simulink library "casper_library_scopes"  (Simulink 7.4)
settings: Solver=ode45  SolverMode=SingleTasking  StartTime=0.0  StopTime=10.0  RelTol=1e-3
libraries: xbsIndex_r4 x369, xps_library x28, casper_library_misc x12, casper_library_scopes x4, simulink x1
(part 2 of 4)

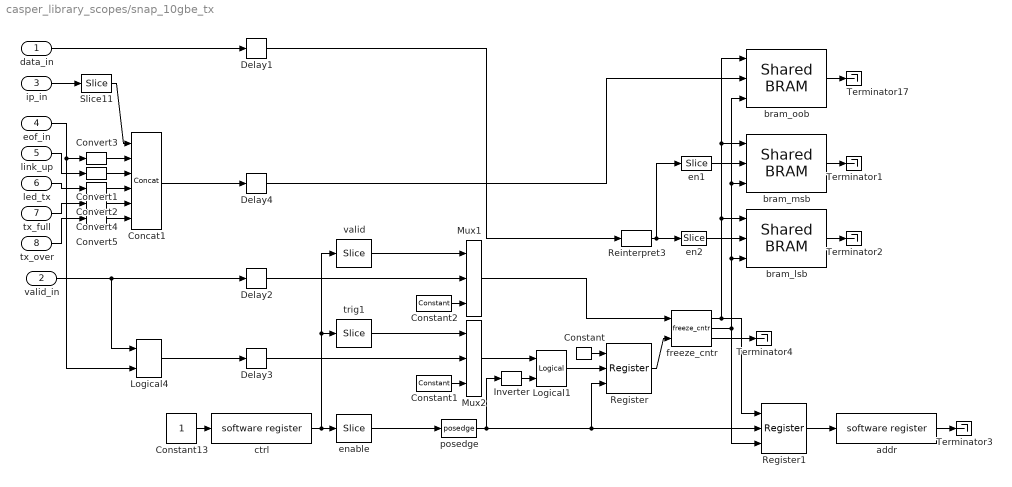
== system casper_library_scopes/snap_10gbe_tx ==
  data_in : Inport  OutDataType=sfix(16)  OutScaling=2^0
  valid_in : Inport  Port=2  OutDataType=sfix(16)  OutScaling=2^0
  ip_in : Inport  Port=3  OutDataType=sfix(16)  OutScaling=2^0
  eof_in : Inport  Port=4  OutDataType=sfix(16)  OutScaling=2^0
  link_up : Inport  Port=5  OutDataType=sfix(16)  OutScaling=2^0
  led_tx : Inport  Port=6  OutDataType=sfix(16)  OutScaling=2^0
  tx_full : Inport  Port=7  OutDataType=sfix(16)  OutScaling=2^0
  tx_over : Inport  Port=8  OutDataType=sfix(16)  OutScaling=2^0
  Concat1 : xbsIndex_r4/Concat  num_inputs=6  dbl_ovrd=off  block_type=concat
      settings: block_version=10.1.3
  Constant : xbsIndex_r4/Constant  arith_type=Boolean  const=1  n_bits=1  bin_pt=0  explicit_period=on  period=1  equ=P=C  opselect=C  inp2=PCIN>>17  opr=+  inp1=P  carry=CIN  dbl_ovrd=off  block_type=constant
  Constant1 : xbsIndex_r4/Constant  arith_type=Boolean  const=1  n_bits=1  bin_pt=0  explicit_period=on  period=1  equ=P=C  opselect=C  inp2=PCIN>>17  opr=+  inp1=P  carry=CIN  dbl_ovrd=off  block_type=constant
  Constant13 : Constant  OutDataType=sfix(16)  OutScaling=2^0
  Constant2 : xbsIndex_r4/Constant  arith_type=Boolean  const=1  n_bits=1  bin_pt=0  explicit_period=on  period=1  equ=P=C  opselect=C  inp2=PCIN>>17  opr=+  inp1=P  carry=CIN  dbl_ovrd=off  block_type=constant
  Convert{1..5} (5 alike) : xbsIndex_r4/Convert  arith_type=Unsigned  n_bits=1  bin_pt=0  quantization=Truncate  overflow=Wrap  latency=0  dbl_ovrd=off  pipeline=off  block_type=convert
      settings: xl_area=[0, 0, 0, 0, 0, 0, 0]  block_version=10.1.3
  Delay{1..4} (4 alike) : xbsIndex_r4/Delay  en=off  latency=2  dbl_ovrd=off  reg_retiming=on  block_type=delay
      settings: xl_area=[0, 0, 0, 0, 0, 0, 0]
  Inverter : xbsIndex_r4/Inverter  en=off  latency=0  dbl_ovrd=off  block_type=inv
      settings: xl_area=[0, 0, 0, 0, 0, 0, 0]
  Logical1 : xbsIndex_r4/Logical  logical_function=AND  inputs=2  en=off  latency=0  precision=Full  arith_type=Unsigned  n_bits=8  bin_pt=2  align_bp=on  dbl_ovrd=off  block_type=logical
      settings: xl_area=[0, 0, 0, 0, 0, 0, 0]
  Logical4 : xbsIndex_r4/Logical  logical_function=AND  inputs=2  en=off  latency=0  precision=Full  arith_type=Unsigned  n_bits=8  bin_pt=2  align_bp=on  dbl_ovrd=off  block_type=logical
      settings: xl_area=[0, 0, 0, 0, 0, 0, 0]
  Mux1 : xbsIndex_r4/Mux  inputs=2  en=off  latency=0  precision=Full  arith_type="Signed  (2's comp)"  n_bits=8  bin_pt=2  quantization=Truncate  overflow=Wrap  dbl_ovrd=off  block_type=mux
      settings: xl_area=[0, 0, 0, 0, 0, 0, 0]
  Mux2 : xbsIndex_r4/Mux  inputs=2  en=off  latency=0  precision=Full  arith_type="Signed  (2's comp)"  n_bits=8  bin_pt=2  quantization=Truncate  overflow=Wrap  dbl_ovrd=off  block_type=mux
      settings: xl_area=[0, 0, 0, 0, 0, 0, 0]
  Register : xbsIndex_r4/Register  init=0  rst=on  en=on  dbl_ovrd=off  block_type=register
      settings: xl_area=[0, 0, 0, 0, 0, 0, 0]
  Register1 : xbsIndex_r4/Register  init=0  rst=on  en=on  dbl_ovrd=off  block_type=register
      settings: xl_area=[0, 0, 0, 0, 0, 0, 0]
  Reinterpret3 : xbsIndex_r4/Reinterpret  force_arith_type=on  arith_type=Unsigned  force_bin_pt=on  bin_pt=0  block_type=reinterpret
      settings: infoedit="Changes signal type without altering the binary representation.   You can changed the signal between signed and unsigned, and relocate the binary point.<P><P>Hardware notes: In hardware this block costs nothing.<P><P>Example:  Suppose the input is 6 bits wide, signed, with 2 fractional bits, and the output is forced to unsigned with 0 fractional bits.  Then an input of -2.0 (1110.00 in binary 2's complement) becomes an output of 56 (111000 in binary)."  block_version=10.1.3
  Slice11 : xbsIndex_r4/Slice  nbits=32-5  boolean_output=off  mode=Lower Bit Location + Width  bit1=0  base1=MSB of Input  bit0=0  base0=LSB of Input  dbl_ovrd=off  block_type=slice
      settings: infoedit="Extracts a given range of bits from each input sample and presents it at the output.  The output type is ordinarily unsigned with binary point at zero, but can be Boolean when the slice is one bit wide.<P><P>Hardware notes: In hardware this block costs nothing."  block_version=10.1.3
  Terminator{1..4,17} (5 alike) : Terminator
  addr : xps_library/software register  Tag=xps:sw_reg  SystemSampleTime=-1  io_dir=To Processor  arith_type=Unsigned  bitwidth=32  bin_pt=0  sample_period=1  gw_name=casper_library_scopes_snap_10gbe_tx_addr_user_data_in
      link override convert: arith_type=Unsigned  n_bits=32  bin_pt=0
  bram_lsb : xps_library/Shared BRAM  Tag=xps:bram  SystemSampleTime=-1  arith_type=Unsigned  addr_width=11  data_width=32  data_bin_pt=0  init_vals=0  sample_rate=1
      link override b_2x_8a_r310b_snap_xaui_tx0_bram_lsb_data_out: arith_type=Unsigned
      link override convert_din: arith_type=Unsigned
      link override mem/sim_data_in: arith_type=Unsigned
      link override r_10gbe_demo_snap_gbe0_tx_bram_lsb_data_out: arith_type=Unsigned
      link override r_10gbe_test_snap_gbe0_tx_bram_lsb_data_out: arith_type=Unsigned
      link override r_10gbe_test_snap_xaui_tx_bram_lsb_data_out: arith_type=Unsigned
      link override r_2x_8a_r310b_snap_xaui_tx0_bram_lsb_data_out: arith_type=Unsigned
      link override r_2x_8a_r311a_snap_xaui_tx0_bram_lsb_data_out: arith_type=Unsigned
      link override r_2x_8a_r311b_snap_xaui_tx0_bram_lsb_data_out: arith_type=Unsigned
  bram_msb : xps_library/Shared BRAM  Tag=xps:bram  SystemSampleTime=-1  arith_type=Unsigned  addr_width=11  data_width=32  data_bin_pt=0  init_vals=0  sample_rate=1
      link override b_2x_8a_r310b_snap_xaui_tx0_bram_msb_data_out: arith_type=Unsigned
      link override convert_din: arith_type=Unsigned
      link override mem/sim_data_in: arith_type=Unsigned
      link override r_10gbe_demo_snap_gbe0_tx_bram_msb_data_out: arith_type=Unsigned
      link override r_10gbe_test_snap_gbe0_tx_bram_msb_data_out: arith_type=Unsigned
      link override r_10gbe_test_snap_xaui_tx_bram_msb_data_out: arith_type=Unsigned
      link override r_2x_8a_r310b_snap_xaui_tx0_bram_msb_data_out: arith_type=Unsigned
      link override r_2x_8a_r311a_snap_xaui_tx0_bram_msb_data_out: arith_type=Unsigned
      link override r_2x_8a_r311b_snap_xaui_tx0_bram_msb_data_out: arith_type=Unsigned
  bram_oob : xps_library/Shared BRAM  Tag=xps:bram  SystemSampleTime=-1  arith_type=Unsigned  addr_width=11  data_width=32  data_bin_pt=0  init_vals=0  sample_rate=1
      link override b_2x_8a_r310b_snap_xaui_tx0_bram_oob_data_out: arith_type=Unsigned
      link override convert_din: arith_type=Unsigned
      link override mem/sim_data_in: arith_type=Unsigned
      link override r_10gbe_demo_snap_gbe0_tx_bram_oob_data_out: arith_type=Unsigned
      link override r_10gbe_test_snap_gbe0_tx_bram_oob_data_out: arith_type=Unsigned
      link override r_10gbe_test_snap_xaui_tx_bram_oob_data_out: arith_type=Unsigned
      link override r_2x_8a_r310b_snap_xaui_tx0_bram_oob_data_out: arith_type=Unsigned
      link override r_2x_8a_r311a_snap_xaui_tx0_bram_oob_data_out: arith_type=Unsigned
      link override r_2x_8a_r311b_snap_xaui_tx0_bram_oob_data_out: arith_type=Unsigned
  ctrl : xps_library/software register  Tag=xps:sw_reg  SystemSampleTime=-1  io_dir=From Processor  arith_type=Unsigned  bitwidth=32  bin_pt=0  sample_period=1  gw_name=casper_library_scopes_snap_10gbe_tx_ctrl_user_data_out
      link override b_2x_8a_r310b_snap_xaui_tx0_ctrl_user_data_out: arith_type=Unsigned  n_bits=32  bin_pt=0  period=1
      link override r_10gbe_demo_snap_gbe0_tx_ctrl_user_data_out: arith_type=Unsigned  n_bits=32  bin_pt=0  period=1
      link override r_10gbe_test_snap_gbe0_tx_ctrl_user_data_out: arith_type=Unsigned  n_bits=32  bin_pt=0  period=1
      link override r_10gbe_test_snap_xaui_tx_ctrl_user_data_out: arith_type=Unsigned  n_bits=32  bin_pt=0  period=1
      link override r_2x_8a_r310b_snap_xaui_tx0_ctrl_user_data_out: arith_type=Unsigned  n_bits=32  bin_pt=0  period=1
      link override r_2x_8a_r311a_snap_xaui_tx0_ctrl_user_data_out: arith_type=Unsigned  n_bits=32  bin_pt=0  period=1
      link override r_2x_8a_r311b_snap_xaui_tx0_ctrl_user_data_out: arith_type=Unsigned  n_bits=32  bin_pt=0  period=1
  en1 : xbsIndex_r4/Slice  nbits=32  boolean_output=off  mode=Lower Bit Location + Width  bit1=0  base1=LSB of Input  bit0=32  base0=LSB of Input  dbl_ovrd=off  block_type=slice
      settings: infoedit="Extracts a given range of bits from each input sample and presents it at the output.  The output type is ordinarily unsigned with binary point at zero, but can be Boolean when the slice is one bit wide.<P><P>Hardware notes: In hardware this block costs nothing."  block_version=10.1.3
  en2 : xbsIndex_r4/Slice  nbits=32  boolean_output=off  mode=Lower Bit Location + Width  bit1=0  base1=LSB of Input  bit0=0  base0=LSB of Input  dbl_ovrd=off  block_type=slice
      settings: infoedit="Extracts a given range of bits from each input sample and presents it at the output.  The output type is ordinarily unsigned with binary point at zero, but can be Boolean when the slice is one bit wide.<P><P>Hardware notes: In hardware this block costs nothing."  block_version=10.1.3
  enable : xbsIndex_r4/Slice  nbits=1  boolean_output=on  mode=Lower Bit Location + Width  bit1=0  base1=LSB of Input  bit0=0  base0=LSB of Input  dbl_ovrd=off  block_type=slice
      settings: infoedit="Extracts a given range of bits from each input sample and presents it at the output.  The output type is ordinarily unsigned with binary point at zero, but can be Boolean when the slice is one bit wide.<P><P>Hardware notes: In hardware this block costs nothing."  block_version=10.1.3
  freeze_cntr : casper_library_misc/freeze_cntr  SystemSampleTime=-1  CounterBits=nsamples
  posedge : casper_library_misc/posedge  Tag=Rising Edge Detector  SystemSampleTime=-1
  trig1 : xbsIndex_r4/Slice  nbits=1  boolean_output=on  mode=Lower Bit Location + Width  bit1=0  base1=LSB of Input  bit0=1  base0=LSB of Input  dbl_ovrd=off  block_type=slice
      settings: infoedit="Extracts a given range of bits from each input sample and presents it at the output.  The output type is ordinarily unsigned with binary point at zero, but can be Boolean when the slice is one bit wide.<P><P>Hardware notes: In hardware this block costs nothing."  block_version=10.1.3
  valid : xbsIndex_r4/Slice  nbits=1  boolean_output=on  mode=Lower Bit Location + Width  bit1=0  base1=LSB of Input  bit0=2  base0=LSB of Input  dbl_ovrd=off  block_type=slice
      settings: infoedit="Extracts a given range of bits from each input sample and presents it at the output.  The output type is ordinarily unsigned with binary point at zero, but can be Boolean when the slice is one bit wide.<P><P>Hardware notes: In hardware this block costs nothing."  block_version=10.1.3
  wires:
  freeze_cntr/3 -> Terminator4/1
  addr/1 -> Terminator3/1
  bram_lsb/1 -> Terminator2/1
  bram_msb/1 -> Terminator1/1
  bram_oob/1 -> Terminator17/1
  Convert5/1 -> Concat1/6
  Convert4/1 -> Concat1/5
  Convert2/1 -> Concat1/4
  Convert1/1 -> Concat1/3
  Convert3/1 -> Concat1/2
  tx_over/1 -> Convert5/1
  tx_full/1 -> Convert4/1
  led_tx/1 -> Convert2/1
  link_up/1 -> Convert1/1
  eof_in/1 -> Logical4/2, Convert3/1
  Delay3/1 -> Mux2/2
  Delay2/1 -> Mux1/2
  valid_in/1 -> Logical4/1, Delay2/1
  Logical4/1 -> Delay3/1
  Delay4/1 -> bram_oob/2
  Delay1/1 -> Reinterpret3/1
  ip_in/1 -> Slice11/1
  data_in/1 -> Delay1/1
  Concat1/1 -> Delay4/1
  Slice11/1 -> Concat1/1
  freeze_cntr/1 -> bram_lsb/1, bram_msb/1, bram_oob/1, Register1/1
  Register/1 -> freeze_cntr/2
  Mux2/1 -> Logical1/1
  Inverter/1 -> Logical1/2
  Logical1/1 -> Register/2
  valid/1 -> Mux1/1
  trig1/1 -> Mux2/1
  Register1/1 -> addr/1
  Constant2/1 -> Mux1/3
  Mux1/1 -> freeze_cntr/1
  Constant1/1 -> Mux2/3
  Constant/1 -> Register/1
  posedge/1 -> Inverter/1, Register1/2, Register/3
  ctrl/1 -> trig1/1, valid/1, enable/1
  Constant13/1 -> ctrl/1
  freeze_cntr/2 -> bram_lsb/3, bram_msb/3, bram_oob/3, Register1/3
  enable/1 -> posedge/1
  Reinterpret3/1 -> en1/1, en2/1
  en1/1 -> bram_msb/2
  en2/1 -> bram_lsb/2

== system casper_library_scopes/snap_32n ==
  trig : Inport
  din : Inport  Port=2
  Constant : Constant  Value=0  OutDataType=sfix(16)  OutScaling=2^0
  read_freeze : xps_library/software register  Tag=xps:sw_reg  SystemSampleTime=-1  io_dir=From Processor  arith_type=Unsigned  bitwidth=32  bin_pt=0  sample_period=1  gw_name=casper_library_scopes_snap_32n_read_freeze_user_data_out
      link override adc_tb_interleaved2_snap_32n_read_freeze_user_data_out: arith_type=Unsigned  n_bits=32  bin_pt=0  period=1
      link override adc_tb_interleaved_snap_32n_read_freeze_user_data_out: arith_type=Unsigned  n_bits=32  bin_pt=0  period=1
  sc0 : casper_library_scopes/sc  SystemSampleTime=-1  nsamples=11  offset=0
      link override bram/adc_tb_interleaved2_snap_32n_sc0_bram_data_out: arith_type=Unsigned
      link override bram/adc_tb_interleaved_snap_32n_sc0_bram_data_out: arith_type=Unsigned
      link override bram/convert_din: arith_type=Unsigned
      link override bram/mem/sim_data_in: arith_type=Unsigned
  sc1 : casper_library_scopes/sc  SystemSampleTime=-1  nsamples=11  offset=32
      link override bram/adc_tb_interleaved2_snap_32n_sc1_bram_data_out: arith_type=Unsigned
      link override bram/adc_tb_interleaved_snap_32n_sc1_bram_data_out: arith_type=Unsigned
      link override bram/convert_din: arith_type=Unsigned
      link override bram/mem/sim_data_in: arith_type=Unsigned
  sc2 : casper_library_scopes/sc  SystemSampleTime=-1  nsamples=11  offset=64
      link override bram/adc_tb_interleaved2_snap_32n_sc2_bram_data_out: arith_type=Unsigned
      link override bram/adc_tb_interleaved_snap_32n_sc2_bram_data_out: arith_type=Unsigned
      link override bram/convert_din: arith_type=Unsigned
      link override bram/mem/sim_data_in: arith_type=Unsigned
  sc3 : casper_library_scopes/sc  SystemSampleTime=-1  nsamples=11  offset=96
      link override bram/adc_tb_interleaved2_snap_32n_sc3_bram_data_out: arith_type=Unsigned
      link override bram/adc_tb_interleaved_snap_32n_sc3_bram_data_out: arith_type=Unsigned
      link override bram/convert_din: arith_type=Unsigned
      link override bram/mem/sim_data_in: arith_type=Unsigned
  wires:
  Constant/1 -> read_freeze/1
  trig/1 -> sc0/2, sc1/2, sc2/2, sc3/2
  din/1 -> sc0/1, sc1/1, sc2/1, sc3/1
  read_freeze/1 -> sc0/3, sc1/3, sc2/3, sc3/3

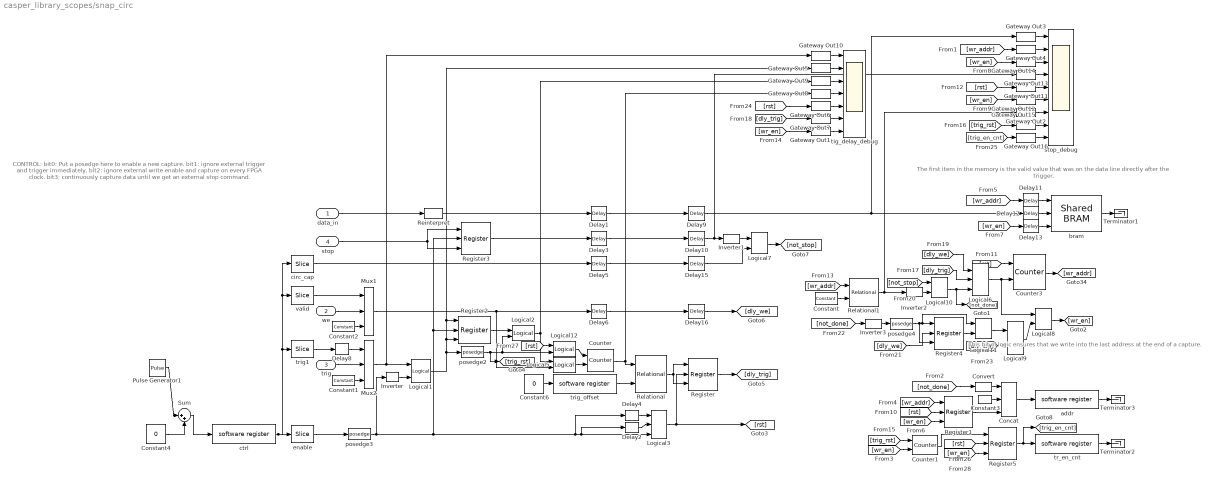
== system casper_library_scopes/snap_circ ==
  note: This bit of logic ensures that we
      | write into the last address
      | at the end of a capture.
  note: The first item in the memory
      | is the valid value that was on the
      | data line directly after the trigger.
  note: CONTROL:
      | bit0: Put a posedge here to enable a new capture.
      | bit1: ignore external trigger and trigger immediately.
      | bit2: ignore external write enable and capture on every FPGA clock.
      | bit3: continuously capture data until we get an external stop command.
  data_in : Inport  OutDataType=sfix(16)  OutScaling=2^0
  we : Inport  Port=2  OutDataType=sfix(16)  OutScaling=2^0
  trig : Inport  Port=3  OutDataType=sfix(16)  OutScaling=2^0
  stop : Inport  Port=4  OutDataType=sfix(16)  OutScaling=2^0
  Concat : xbsIndex_r4/Concat  num_inputs=3  dbl_ovrd=off  block_type=concat
      settings: block_version=10.1.3
  Constant : xbsIndex_r4/Constant  arith_type=Unsigned  const=(2^nsamples)-1  n_bits=nsamples  bin_pt=0  explicit_period=on  period=1  equ=P=C  opselect=C  inp2=PCIN>>17  opr=+  inp1=P  carry=CIN  dbl_ovrd=off  block_type=constant
  Constant1 : xbsIndex_r4/Constant  arith_type=Boolean  const=1  n_bits=1  bin_pt=0  explicit_period=on  period=1  equ=P=C  opselect=C  inp2=PCIN>>17  opr=+  inp1=P  carry=CIN  dbl_ovrd=off  block_type=constant
  Constant2 : xbsIndex_r4/Constant  arith_type=Boolean  const=1  n_bits=1  bin_pt=0  explicit_period=on  period=1  equ=P=C  opselect=C  inp2=PCIN>>17  opr=+  inp1=P  carry=CIN  dbl_ovrd=off  block_type=constant
  Constant3 : xbsIndex_r4/Constant  arith_type=Unsigned  const=0  n_bits=32-nsamples-1  bin_pt=0  explicit_period=on  period=1  equ=P=C  opselect=C  inp2=PCIN>>17  opr=+  inp1=P  carry=CIN  dbl_ovrd=off  block_type=constant
  Constant4 : Constant  Value=0  OutDataType=sfix(16)  OutScaling=2^0
  Constant6 : Constant  Value=0  OutDataType=sfix(16)  OutScaling=2^0
  Convert : xbsIndex_r4/Convert  arith_type=Unsigned  n_bits=1  bin_pt=0  quantization=Truncate  overflow=Wrap  latency=0  dbl_ovrd=off  pipeline=off  block_type=convert
      settings: block_version=10.1.3
  Counter : xbsIndex_r4/Counter  cnt_type=Free Running  cnt_to=Inf  operation=Up  start_count=0  cnt_by_val=1  arith_type=Unsigned  n_bits=32  bin_pt=0  load_pin=off  rst=on  en=on  explicit_period=on  period=1  dbl_ovrd=off  use_behavioral_HDL=off  implementation=Fabric  use_rpm=on  block_type=counter
      settings: xl_area=[0, 0, 0, 0, 0, 0, 0]
  Counter1 : xbsIndex_r4/Counter  cnt_type=Free Running  cnt_to=Inf  operation=Up  start_count=0  cnt_by_val=1  arith_type=Unsigned  n_bits=32  bin_pt=0  load_pin=off  rst=on  en=on  explicit_period=on  period=1  dbl_ovrd=off  use_behavioral_HDL=off  implementation=Fabric  use_rpm=on  block_type=counter
      settings: xl_area=[0, 0, 0, 0, 0, 0, 0]
  Counter3 : xbsIndex_r4/Counter  cnt_type=Free Running  cnt_to=1  operation=Up  start_count=0  cnt_by_val=1  arith_type=Unsigned  n_bits=nsamples  bin_pt=0  load_pin=off  rst=on  en=on  explicit_period=on  period=1  dbl_ovrd=off  use_behavioral_HDL=off  implementation=Fabric  use_rpm=on  block_type=counter
      settings: xl_area=[0, 0, 0, 0, 0, 0, 0]
  Delay{1,3..6,9..13,15..16} (12 alike) : xbsIndex_r4/Delay  en=off  latency=1  dbl_ovrd=off  reg_retiming=on  block_type=delay
      settings: xl_area=[0, 0, 0, 0, 0, 0, 0]
  Delay2 : xbsIndex_r4/Delay  en=off  latency=2  dbl_ovrd=off  reg_retiming=on  block_type=delay
      settings: xl_area=[0, 0, 0, 0, 0, 0, 0]
  Delay8 : xbsIndex_r4/Delay  en=off  latency=3  dbl_ovrd=off  reg_retiming=on  block_type=delay
      settings: xl_area=[0, 0, 0, 0, 0, 0, 0]
  Gateway Out{1..16} (16 alike) : xbsIndex_r4/Gateway Out  hdl_port=off  timing_constraint=None  locs_specified=off  LOCs={}  block_type=gatewayout
      settings: infoedit="Gateway out block.  Converts Xilinx fixed point inputs into ouputs of type Simulink integer, double, or fixed point.<P><P>Hardware notes:  In hardware these blocks become top level output ports or are discarded, depending on how they are configured."  xl_area=[0, 0, 0, 0, 0, 0, 0]  block_version=10.1.3
  Inverter{,1..3} (4 alike) : xbsIndex_r4/Inverter  en=off  latency=0  dbl_ovrd=off  block_type=inv
      settings: xl_area=[0, 0, 0, 0, 0, 0, 0]
  Logical{1,5,7,9} (4 alike) : xbsIndex_r4/Logical  logical_function=AND  inputs=2  en=off  latency=0  precision=Full  arith_type=Unsigned  n_bits=8  bin_pt=2  align_bp=on  dbl_ovrd=off  block_type=logical
      settings: xl_area=[0, 0, 0, 0, 0, 0, 0]
  Logical{2,8,10..12} (5 alike) : xbsIndex_r4/Logical  logical_function=OR  inputs=2  en=off  latency=0  precision=Full  arith_type=Unsigned  n_bits=8  bin_pt=2  align_bp=on  dbl_ovrd=off  block_type=logical
      settings: xl_area=[0, 0, 0, 0, 0, 0, 0]
  Logical3 : xbsIndex_r4/Logical  logical_function=OR  inputs=3  en=off  latency=0  precision=Full  arith_type=Unsigned  n_bits=8  bin_pt=2  align_bp=on  dbl_ovrd=off  block_type=logical
      settings: xl_area=[0, 0, 0, 0, 0, 0, 0]
  Logical6 : xbsIndex_r4/Logical  logical_function=AND  inputs=3  en=off  latency=0  precision=Full  arith_type=Unsigned  n_bits=8  bin_pt=2  align_bp=on  dbl_ovrd=off  block_type=logical
      settings: xl_area=[0, 0, 0, 0, 0, 0, 0]
  Mux1 : xbsIndex_r4/Mux  inputs=2  en=off  latency=0  precision=Full  arith_type="Signed  (2's comp)"  n_bits=8  bin_pt=2  quantization=Truncate  overflow=Wrap  dbl_ovrd=off  block_type=mux
      settings: xl_area=[0, 0, 0, 0, 0, 0, 0]
  Mux2 : xbsIndex_r4/Mux  inputs=2  en=off  latency=0  precision=Full  arith_type="Signed  (2's comp)"  n_bits=8  bin_pt=2  quantization=Truncate  overflow=Wrap  dbl_ovrd=off  block_type=mux
      settings: xl_area=[0, 0, 0, 0, 0, 0, 0]
  Pulse Generator1 : DiscretePulseGenerator  Amplitude=1  Period=2^(nsamples+2)  PulseWidth=2  PhaseDelay=0  SampleTime=1
  Register{,1..5} (6 alike) : xbsIndex_r4/Register  init=0  rst=on  en=on  dbl_ovrd=off  block_type=register
      settings: xl_area=[0, 0, 0, 0, 0, 0, 0]
  Reinterpret : xbsIndex_r4/Reinterpret  force_arith_type=on  arith_type=Unsigned  force_bin_pt=on  bin_pt=0  block_type=reinterpret
      settings: infoedit="Changes signal type without altering the binary representation.   You can changed the signal between signed and unsigned, and relocate the binary point.<P><P>Hardware notes: In hardware this block costs nothing.<P><P>Example:  Suppose the input is 6 bits wide, signed, with 2 fractional bits, and the output is forced to unsigned with 0 fractional bits.  Then an input of -2.0 (1110.00 in binary 2's complement) becomes an output of 56 (111000 in binary)."  block_version=10.1.3
  Relational : xbsIndex_r4/Relational  mode=a>b  en=off  latency=0  dbl_ovrd=off  block_type=relational
      settings: xl_area=[0, 0, 0, 0, 0, 0, 0]  block_version=10.1.3
  Relational1 : xbsIndex_r4/Relational  mode=a>=b  en=off  latency=0  dbl_ovrd=off  block_type=relational
      settings: xl_area=[0, 0, 0, 0, 0, 0, 0]  block_version=10.1.3
  Sum : Sum  Inputs=|++  OutDataType=sfix(16)  OutScaling=2^0
  Terminator1 : Terminator
  Terminator2 : Terminator
  Terminator3 : Terminator
  addr : xps_library/software register  Tag=xps:sw_reg  SystemSampleTime=-1  io_dir=To Processor  arith_type=Unsigned  bitwidth=32  bin_pt=0  sample_period=1  gw_name=casper_library_scopes_snap_circ_addr_user_data_in
      link override convert: arith_type=Unsigned  n_bits=32  bin_pt=0
  bram : xps_library/Shared BRAM  Tag=xps:bram  SystemSampleTime=-1  arith_type=Unsigned  addr_width=10  data_width=32  data_bin_pt=0  init_vals=0  sample_rate=1
      link override convert_din: arith_type=Unsigned
      link override mem/sim_data_in: arith_type=Unsigned
      link override r_4f_2x_16a_r322d_snap_descramble0_bram_data_out: arith_type=Unsigned
      link override test_snap2_10_1_snap_circ_bram_lsb_data_out: arith_type=Unsigned
      link override test_snap_circ_snap_circ_bram_data_out: arith_type=Unsigned
  circ_cap : xbsIndex_r4/Slice  nbits=1  boolean_output=on  mode=Lower Bit Location + Width  bit1=0  base1=LSB of Input  bit0=3  base0=LSB of Input  dbl_ovrd=off  block_type=slice
      settings: infoedit="Extracts a given range of bits from each input sample and presents it at the output.  The output type is ordinarily unsigned with binary point at zero, but can be Boolean when the slice is one bit wide.<P><P>Hardware notes: In hardware this block costs nothing."  block_version=10.1.3
  ctrl : xps_library/software register  Tag=xps:sw_reg  SystemSampleTime=-1  io_dir=From Processor  arith_type=Unsigned  bitwidth=32  bin_pt=0  sample_period=1  gw_name=casper_library_scopes_snap_circ_ctrl_user_data_out
      link override r_4f_2x_16a_r322d_snap_descramble0_ctrl_user_data_out: arith_type=Unsigned  n_bits=32  bin_pt=0  period=1
      link override test_snap2_10_1_snap_circ_ctrl_user_data_out: arith_type=Unsigned  n_bits=32  bin_pt=0  period=1
      link override test_snap_circ_snap_circ_ctrl_user_data_out: arith_type=Unsigned  n_bits=32  bin_pt=0  period=1
  enable : xbsIndex_r4/Slice  nbits=1  boolean_output=on  mode=Lower Bit Location + Width  bit1=0  base1=LSB of Input  bit0=0  base0=LSB of Input  dbl_ovrd=off  block_type=slice
      settings: infoedit="Extracts a given range of bits from each input sample and presents it at the output.  The output type is ordinarily unsigned with binary point at zero, but can be Boolean when the slice is one bit wide.<P><P>Hardware notes: In hardware this block costs nothing."  block_version=10.1.3
  posedge2 : casper_library_misc/posedge  Tag=Rising Edge Detector  SystemSampleTime=-1
  posedge3 : casper_library_misc/posedge  Tag=Rising Edge Detector  SystemSampleTime=-1
  posedge4 : casper_library_misc/posedge  Tag=Rising Edge Detector  SystemSampleTime=-1
  stop_debug : Scope  NumInputPorts=9
      settings: YMin=2.72014e+008~0~0~-5~-5~-5~-5~-5~-5  YMax=3.00648e+008~110~1~5~5~5~5~5~5  SaveName=ScopeData12
  tig_delay_debug : Scope  NumInputPorts=7
      settings: YMin=2.72014e+008~0~0~-5~-5~-5~-5  YMax=3.00648e+008~110~1~5~5~5~5  SaveName=ScopeData16
  tr_en_cnt : xps_library/software register  Tag=xps:sw_reg  SystemSampleTime=-1  io_dir=To Processor  arith_type=Unsigned  bitwidth=32  bin_pt=0  sample_period=1  gw_name=casper_library_scopes_snap_circ_tr_en_cnt_user_data_in
      link override convert: arith_type=Unsigned  n_bits=32  bin_pt=0
  trig1 : xbsIndex_r4/Slice  nbits=1  boolean_output=on  mode=Lower Bit Location + Width  bit1=0  base1=LSB of Input  bit0=1  base0=LSB of Input  dbl_ovrd=off  block_type=slice
      settings: infoedit="Extracts a given range of bits from each input sample and presents it at the output.  The output type is ordinarily unsigned with binary point at zero, but can be Boolean when the slice is one bit wide.<P><P>Hardware notes: In hardware this block costs nothing."  block_version=10.1.3
  trig_offset : xps_library/software register  Tag=xps:sw_reg  SystemSampleTime=-1  io_dir=From Processor  arith_type=Unsigned  bitwidth=32  bin_pt=0  sample_period=1  gw_name=casper_library_scopes_snap_circ_trig_offset_user_data_out
      link override test_snap_circ_snap_circ_trig_offset_user_data_out: arith_type=Unsigned  n_bits=32  bin_pt=0  period=1
  valid : xbsIndex_r4/Slice  nbits=1  boolean_output=on  mode=Lower Bit Location + Width  bit1=0  base1=LSB of Input  bit0=2  base0=LSB of Input  dbl_ovrd=off  block_type=slice
      settings: infoedit="Extracts a given range of bits from each input sample and presents it at the output.  The output type is ordinarily unsigned with binary point at zero, but can be Boolean when the slice is one bit wide.<P><P>Hardware notes: In hardware this block costs nothing."  block_version=10.1.3
  wires:
  Delay6/1 -> Delay16/1
  Delay5/1 -> Delay15/1
  Delay3/1 -> Delay10/1
  Delay1/1 -> Delay9/1
  posedge2/1 -> [trig_rst], Logical12/2, Logical2/2
  [rst] -> Logical12/1
  Logical12/1 -> Counter/1
  Register5/1 -> [trig_en_cnt], tr_en_cnt/1
  [rst] -> Register5/2
  [wr_en] -> Register5/3
  Counter1/1 -> Register5/1
  Gateway Out16/1 -> stop_debug/9
  [trig_en_cnt] -> Gateway Out16/1
  Delay8/1 -> Mux2/1
  [rst] -> Gateway Out6/1
  Register4/1 -> Logical11/2
  Logical11/1 -> Logical9/1
  Logical9/1 -> Logical8/2
  [dly_we] -> Logical9/2
  [dly_we] -> Register4/2
  posedge4/1 -> Logical11/1, Register4/1, Register4/3
  Inverter3/1 -> posedge4/1
  [not_done] -> Inverter3/1
  Logical8/1 -> [wr_en]
  [not_stop] -> Logical10/1
  Logical7/1 -> [not_stop]
  [dly_trig] -> Logical6/2
  [dly_we] -> Logical6/1
  Delay16/1 -> [dly_we]
  [dly_trig] -> Gateway Out7/1
  Register/1 -> [dly_trig]
  [trig_rst] -> Gateway Out15/1
  Gateway Out15/1 -> stop_debug/8
  [trig_rst] -> Counter1/1
  [wr_en] -> Gateway Out1/1
  [wr_addr] -> Relational1/1
  Relational1/1 -> Inverter2/1, Gateway Out2/1
  [rst] -> Gateway Out11/1
  [rst] -> Counter3/1
  [rst] -> Register1/2
  [wr_en] -> Gateway Out12/1
  [wr_en] -> Gateway Out14/1
  [wr_en] -> Delay13/1
  [wr_en] -> Register1/3
  [wr_addr] -> Register1/1
  [wr_en] -> Counter1/2
  [not_done] -> Convert/1
  [wr_addr] -> Gateway Out4/1
  [wr_addr] -> Delay11/1
  Register1/1 -> Concat/3
  Logical5/1 -> Counter/2
  Delay15/1 -> Logical7/2
  Delay10/1 -> Gateway Out13/1, Inverter1/1
  Delay9/1 -> Gateway Out3/1, Delay12/1
  bram/1 -> Terminator1/1
  addr/1 -> Terminator3/1
  tr_en_cnt/1 -> Terminator2/1
  Constant3/1 -> Concat/2
  Convert/1 -> Concat/1
  circ_cap/1 -> Delay5/1
  stop/1 -> Register3/3, Register3/1
  Concat/1 -> addr/1
  Delay13/1 -> bram/3
  Delay12/1 -> bram/2
  Delay11/1 -> bram/1
  Inverter2/1 -> Logical10/2
  Logical10/1 -> [not_done], Logical6/3
  Logical3/1 -> [rst], Register/2
  Gateway Out2/1 -> stop_debug/7
  Gateway Out12/1 -> stop_debug/6
  Gateway Out3/1 -> stop_debug/1
  Gateway Out11/1 -> stop_debug/5
  Gateway Out13/1 -> stop_debug/4
  Gateway Out4/1 -> stop_debug/2
  Gateway Out14/1 -> stop_debug/3
  Inverter1/1 -> Logical7/1
  Register3/1 -> Delay3/1
  Constant/1 -> Relational1/2
  Counter3/1 -> [wr_addr]
  Logical6/1 -> Logical8/1, Counter3/2
  Reinterpret/1 -> Delay1/1
  Gateway Out1/1 -> tig_delay_debug/7
  Gateway Out7/1 -> tig_delay_debug/6
  Gateway Out10/1 -> tig_delay_debug/1
  Gateway Out6/1 -> tig_delay_debug/5
  Gateway Out8/1 -> tig_delay_debug/4
  Gateway Out5/1 -> tig_delay_debug/2
  Gateway Out9/1 -> tig_delay_debug/3
  Delay2/1 -> Logical3/2
  Counter/1 -> Relational/1, Gateway Out8/1
  Logical2/1 -> Gateway Out9/1, Logical5/1
  Relational/1 -> Register/1, Register/3
  trig_offset/1 -> Relational/2
  Constant6/1 -> trig_offset/1
  Delay4/1 -> Logical3/1
  Register2/1 -> Logical2/1
  Logical1/1 -> posedge2/1, Register2/3, Gateway Out5/1, Register2/1
  posedge3/1 -> Register3/2, Register2/2, Logical3/3, Delay2/1, Delay4/1, Inverter/1
  Mux1/1 -> Delay6/1, Logical5/2
  Inverter/1 -> Logical1/2
  Mux2/1 -> Gateway Out10/1, Logical1/1
  Pulse Generator1/1 -> Sum/1
  Sum/1 -> ctrl/1
  Constant4/1 -> Sum/2
  trig/1 -> Mux2/2
  enable/1 -> posedge3/1
  ctrl/1 -> enable/1, circ_cap/1, valid/1, trig1/1
  Constant1/1 -> Mux2/3
  we/1 -> Mux1/2
  Constant2/1 -> Mux1/3
  trig1/1 -> Delay8/1
  valid/1 -> Mux1/1
  data_in/1 -> Reinterpret/1

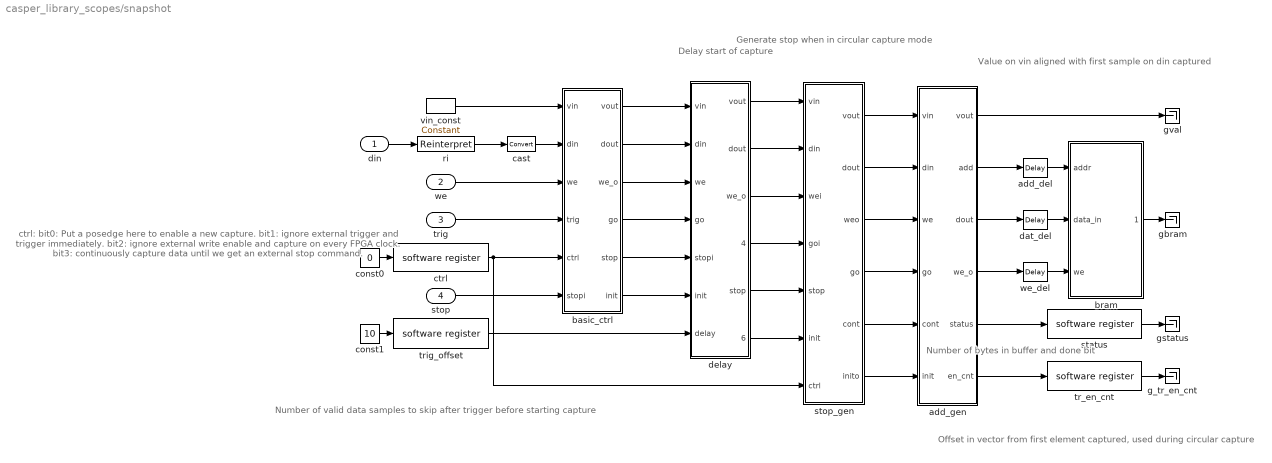
== system casper_library_scopes/snapshot ==
  note: Value on vin
      | aligned with
      | first sample on
      | din captured
  note: Number of valid
      | data samples to
      | skip after trigger
      | before starting
      | capture
  note: Number of
      | bytes in
      | buffer and
      | done bit
  note: Offset in vector
      | from first element
      | captured, used
      | during circular capture
  note: ctrl:
      | bit0: Put a posedge here
      |         to enable a new capture.
      | bit1: ignore external trigger
      |         and trigger immediately.
      | bit2: ignore external write
      |         enable and capture on
      |         every FPGA clock.
      | bit3: continuously capture
      |         data until we get an
      |         external stop command.
  note: Delay start
      | of capture
  note: Generate stop
      | when in circular
      | capture mode
  din : Inport
  we : Inport  Port=2
  trig : Inport  Port=3
  stop : Inport  Port=4
  add_del : xbsIndex_r4/Delay  en=off  latency=1  dbl_ovrd=off  reg_retiming=on  block_type=delay
      settings: block_version=11.4
  add_gen : Subsystem  mask{counter_size=32, increment=4, nsamples=10, burst_size=0, use_dsp48=on}
      mask prompts: counter_size "Address counter size (2^?)"; increment "Address counter increment"; nsamples "Number of samples (2^?)"; burst_size "Burst size (2^?)"; use_dsp48 "dsp48 counter/s"
      mask init:
      | set_param(gcb,'LinkStatus','inactive');
      | if strcmp(use_dsp48,'on'),
      |     set_param([gcb,'/add_gen'],'implementation','DSP48');
      | else
      |     set_param([gcb,'/add_gen'],'implementation','Fabric');
      | end
  basic_ctrl : Subsystem  mask{dram=off, data_width=32}
      mask prompts: data_width "data width"
      mask init:
      | set_param(gcb,'LinkStatus','inactive');
      | set_param([gcb,'/dram_munge'], 'dram', dram);
  bram : Subsystem  Tag=xps:bram  AncestorBlock=xps_library/Shared BRAM  mask{arith_type=Unsigned, addr_width=10, data_width=32, data_bin_pt=0, init_vals=[0:2^10-1], sample_rate=1}
      mask prompts: arith_type "Output Data Type"; addr_width "Address width"; data_width "Data Width"; data_bin_pt "Data Binary Point"; init_vals "Initial 32-bit values (simulation only)"; sample_rate "Sample rate"
      mask init:
      | shared_bram_mask;
      mask StyleString: popup(Unsigned|Signed  (2's comp)),edit,popup(8|16|32|64|128),edit,edit,edit
  cast : xbsIndex_r4/Convert  arith_type=Unsigned  n_bits=32  bin_pt=0  quantization=Truncate  overflow=Wrap  latency=0  dbl_ovrd=off  pipeline=off  block_type=convert
      settings: block_version=11.4
  const0 : Constant  Value=0
  const1 : Constant  Value=10
  ctrl : xps_library/software register  Tag=xps:sw_reg  SystemSampleTime=-1  io_dir=From Processor  arith_type=Unsigned  bitwidth=32  bin_pt=0  sample_period=1  gw_name=casper_library_scopes_snapshot_ctrl_user_data_out
  dat_del : xbsIndex_r4/Delay  en=off  latency=1  dbl_ovrd=off  reg_retiming=on  block_type=delay
      settings: block_version=11.4
  delay : Subsystem  mask{use_dsp48=on, word_size=4}
      mask prompts: use_dsp48 "dsp48 counter/s"; word_size "word byte size?"
      mask init:
      | set_param(gcb,'LinkStatus','inactive');
      | if strcmp(use_dsp48,'on'),
      |     set_param([gcb,'/counter'],'implementation','DSP48');
      | else
      |     set_param([gcb,'/counter'],'implementation','Fabric');
      | end
  g_tr_en_cnt : Terminator
  gbram : Terminator
  gstatus : Terminator
  gval : Terminator
  ri : xbsIndex_r4/Reinterpret  force_arith_type=on  arith_type=Unsigned  force_bin_pt=on  bin_pt=0  block_type=reinterpret
      settings: infoedit="Changes signal type without altering the binary representation.   You can changed the signal between signed and unsigned, and relocate the binary point.<br><br>Hardware notes: In hardware this block costs nothing.<br><br>Example:  Suppose the input is 6 bits wide, signed, with 2 fractional bits, and the output is forced to unsigned with 0 fractional bits.  Then an input of -2.0 (1110.00 in binary 2's complement) becomes an output of 56 (111000 in binary)."
  status : xps_library/software register  Tag=xps:sw_reg  SystemSampleTime=-1  io_dir=To Processor  arith_type=Unsigned  bitwidth=32  bin_pt=0  sample_period=1  gw_name=casper_library_scopes_snapshot_status_user_data_in
  stop_gen : Subsystem
  tr_en_cnt : xps_library/software register  Tag=xps:sw_reg  SystemSampleTime=-1  io_dir=To Processor  arith_type=Unsigned  bitwidth=32  bin_pt=0  sample_period=1  gw_name=casper_library_scopes_snapshot_tr_en_cnt_user_data_in
  trig_offset : xps_library/software register  Tag=xps:sw_reg  SystemSampleTime=-1  io_dir=From Processor  arith_type=Unsigned  bitwidth=32  bin_pt=0  sample_period=1  gw_name=casper_library_scopes_snapshot_trig_offset_user_data_out
  vin_const : xbsIndex_r4/Constant  arith_type=Boolean  const=0  n_bits=16  bin_pt=14  explicit_period=on  period=1  equ=P=C  opselect=C  inp2=PCIN>>17  opr=+  inp1=P  carry=CIN  dbl_ovrd=off  block_type=constant
      settings: block_version=11.4
  we_del : xbsIndex_r4/Delay  en=off  latency=1  dbl_ovrd=off  reg_retiming=on  block_type=delay
      settings: block_version=11.4
  wires:
  din/1 -> ri/1
  ri/1 -> cast/1
  cast/1 -> basic_ctrl/2(din)
  we/1 -> basic_ctrl/3(we)
  trig/1 -> basic_ctrl/4(trig)
  stop/1 -> basic_ctrl/6(stopi)
  const0/1 -> ctrl/1
  ctrl/1 -> basic_ctrl/5(ctrl), stop_gen/7(ctrl)
  const1/1 -> trig_offset/1
  basic_ctrl/1(vout) -> delay/1(vin)
  basic_ctrl/2(dout) -> delay/2(din)
  basic_ctrl/3(we_o) -> delay/3(we)
  basic_ctrl/4(go) -> delay/4(go)
  basic_ctrl/5(stop) -> delay/5(stopi)
  basic_ctrl/6(init) -> delay/6(init)
  trig_offset/1 -> delay/7(delay)
  delay/1(vout) -> stop_gen/1(vin)
  delay/2(dout) -> stop_gen/2(din)
  delay/3(we_o) -> stop_gen/3(wei)
  delay/4(del_go) -> stop_gen/4(goi)
  delay/5(stop) -> stop_gen/5(stop)
  delay/6(del_init) -> stop_gen/6(init)
  tr_en_cnt/1 -> g_tr_en_cnt/1
  stop_gen/1(vout) -> add_gen/1(vin)
  stop_gen/2(dout) -> add_gen/2(din)
  stop_gen/3(weo) -> add_gen/3(we)
  stop_gen/4(go) -> add_gen/4(go)
  stop_gen/5(cont) -> add_gen/5(cont)
  stop_gen/6(inito) -> add_gen/6(init)
  add_gen/5(status) -> status/1
  status/1 -> gstatus/1
  vin_const/1 -> basic_ctrl/1(vin)
  add_gen/1(vout) -> gval/1
  add_gen/6(en_cnt) -> tr_en_cnt/1
  add_gen/2(add) -> add_del/1
  add_gen/3(dout) -> dat_del/1
  add_gen/4(we_o) -> we_del/1
  add_del/1 -> bram/1(addr)
  dat_del/1 -> bram/2(data_in)
  we_del/1 -> bram/3(we)
  bram/1(data_out) -> gbram/1
